simulink model "fluidDynamicSurface_th"  (R2020a)
settings: Solver=VariableStepAuto  StartTime=0.0  StopTime=0  RelTol=1e-3
values from neighbouring files (symbols this model uses):
  angVelBdy = [0 0 0]    [fluidDynamicSurface_ts.m]
  ctrlSurfDefl = (csMin-cSMax).*rand(4,1) + cSMax    [fluidDynamicSurface_ts.m]
  velCMBdy = [1 0 0]    [fluidDynamicSurface_ts.m]
  velWindBdy = repmat([ii; 0; 0],1,4)    [fluidDynamicSurface_ts.m]
undefined symbols (not defined in the file or in its folder): vhcl
libraries: fluidDynamicSurface_cl x1, Copy_of_fluidDynamicSurface_cl x1
settings Model: Creator=mcobb  LastModifiedBy=Ayaz
settings DataIOCC: ReturnWorkspaceOutputs=off
settings DebuggingCC: ArithmeticOperatorsInVariantConditions=warning
settings SFSimCC: CustomCodeUndefinedFunction=UseInterfaceOnly

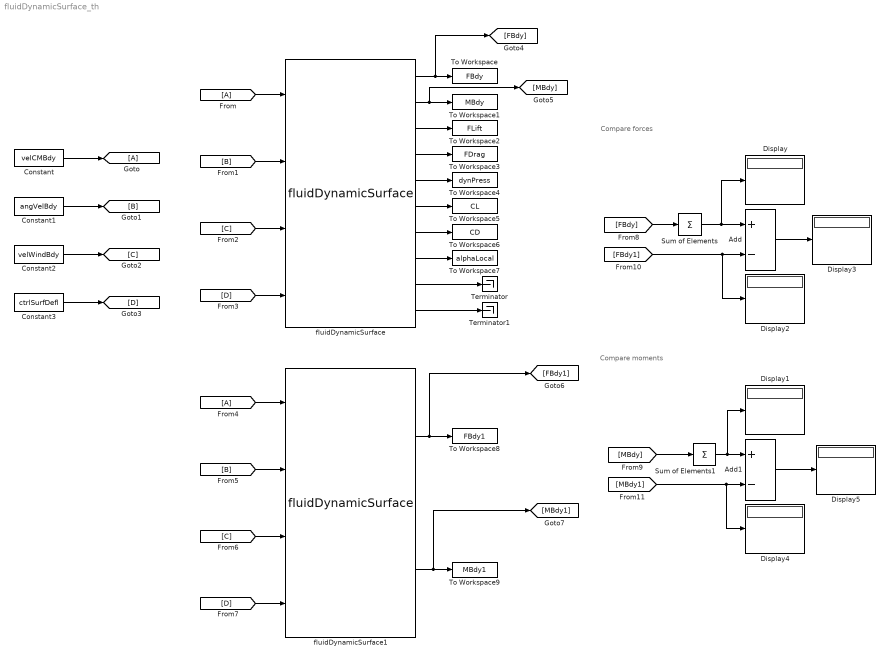
== system fluidDynamicSurface_th ==
  note: Compare moments
  note: Compare forces
  Add : Sum  Inputs=+-
  Add1 : Sum  Inputs=+-
  Constant : Constant  Value=velCMBdy
  Constant1 : Constant  Value=angVelBdy
  Constant2 : Constant  Value=velWindBdy
  Constant3 : Constant  Value=ctrlSurfDefl
  Display{,1..5} (6 alike) : Display
  Sum of Elements : Sum  Inputs=+  CollapseMode=Specified dimension  CollapseDim=2
  Sum of Elements1 : Sum  Inputs=+  CollapseMode=Specified dimension  CollapseDim=2
  Terminator : Terminator
  Terminator1 : Terminator
  To Workspace : ToWorkspace  VariableName=FBdy  SaveFormat=Timeseries  SampleTime=-1
  To Workspace1 : ToWorkspace  VariableName=MBdy  SaveFormat=Timeseries  SampleTime=-1
  To Workspace2 : ToWorkspace  VariableName=FLift  SaveFormat=Timeseries  SampleTime=-1
  To Workspace3 : ToWorkspace  VariableName=FDrag  SaveFormat=Timeseries  SampleTime=-1
  To Workspace4 : ToWorkspace  VariableName=dynPress  SaveFormat=Timeseries  SampleTime=-1
  To Workspace5 : ToWorkspace  VariableName=CL  SaveFormat=Timeseries  SampleTime=-1
  To Workspace6 : ToWorkspace  VariableName=CD  SaveFormat=Timeseries  SampleTime=-1
  To Workspace7 : ToWorkspace  VariableName=alphaLocal  SaveFormat=Timeseries  SampleTime=-1
  To Workspace8 : ToWorkspace  VariableName=FBdy1  SaveFormat=Timeseries  SampleTime=-1
  To Workspace9 : ToWorkspace  VariableName=MBdy1  SaveFormat=Timeseries  SampleTime=-1
  fluidDynamicSurface : fluidDynamicSurface_cl/fluidDynamicSurface  aeroStruct=vhcl.struct('OCT.aeroSurf')  fluidDensity=fluidDensity  fluidMomentArms=vhcl.fluidMomentArms.Value  fluidRefArea=vhcl.fluidRefArea.Value  wingTips=vhcl.wingTipPositions.Value
  fluidDynamicSurface1 : Copy_of_fluidDynamicSurface_cl/fluidDynamicSurface  vcl=vhcl  fluidDensity=fluidDensity  fluidMomentArms=vhcl.fluidMomentArms.Value  fluidRefArea=vhcl.fluidRefArea.Value  wingTips=vhcl.wingTipPositions.Value
  wires:
  fluidDynamicSurface/1 -> [FBdy], To Workspace/1
  Constant/1 -> [A]
  Constant1/1 -> [B]
  Constant2/1 -> [C]
  fluidDynamicSurface/3 -> To Workspace2/1
  fluidDynamicSurface/4 -> To Workspace3/1
  fluidDynamicSurface/2 -> [MBdy], To Workspace1/1
  fluidDynamicSurface/5 -> To Workspace4/1
  fluidDynamicSurface/6 -> To Workspace5/1
  fluidDynamicSurface/7 -> To Workspace6/1
  fluidDynamicSurface/8 -> To Workspace7/1
  Constant3/1 -> [D]
  fluidDynamicSurface/9 -> Terminator/1
  [A] -> fluidDynamicSurface/1
  [B] -> fluidDynamicSurface/2
  [C] -> fluidDynamicSurface/3
  [D] -> fluidDynamicSurface/4
  [C] -> fluidDynamicSurface1/3
  [D] -> fluidDynamicSurface1/4
  [B] -> fluidDynamicSurface1/2
  [A] -> fluidDynamicSurface1/1
  fluidDynamicSurface/10 -> Terminator1/1
  fluidDynamicSurface1/1 -> [FBdy1], To Workspace8/1
  fluidDynamicSurface1/2 -> [MBdy1], To Workspace9/1
  [FBdy] -> Sum of Elements/1
  [MBdy] -> Sum of Elements1/1
  Sum of Elements/1 -> Display/1, Add/1
  [FBdy1] -> Display2/1, Add/2
  Add/1 -> Display3/1
  Sum of Elements1/1 -> Display1/1, Add1/1
  Add1/1 -> Display5/1
  [MBdy1] -> Display4/1, Add1/2
